simulink subsystem "LRLM_ECU"  (R2021a)
settings: Solver=VariableStepAuto  StartTime=0.0  StopTime=10.0  RelTol=1e-3
libraries: LRLM x4, simulink x2, BCM x1
settings Model: Creator=Sai229  LastModifiedBy=Sai229

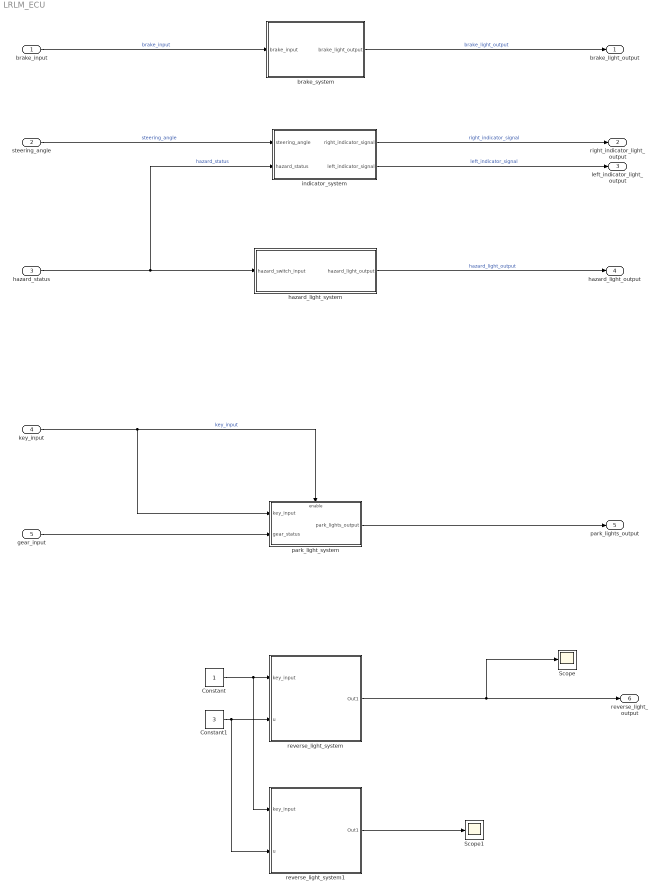
== system LRLM_ECU ==
  brake_input : Inport
  steering_angle : Inport  Port=2
  hazard_status : Inport  Port=3
  key_input : Inport  Port=4
  gear_input : Inport  Port=5
  Constant : Constant
  Constant1 : Constant  Value=3
  Scope : Scope
  Scope1 : Scope
  brake_system : Subsystem  TreatAsAtomicUnit=on
      mask Display: disp("Brake System");
  hazard_light_system : Subsystem
  indicator_system : Subsystem  TreatAsAtomicUnit=on
  park_light_system : Subsystem
  reverse_light_system : Subsystem  TreatAsAtomicUnit=on  mask{Parameter1=0, time_period=1}
      mask prompts: time_period "Enter the time period for blinking the light"
  reverse_light_system1 : Subsystem
      mask help: Simulink:masks:GenSFuncDesc_MD
      mask Help: eval('feval(''rtwprivate'',''rtwhelpview'',''rtw_sfcn_block'')');
  brake_light_output : Outport
  right_indicator_light_output : Outport  Port=2
  left_indicator_light_output : Outport  Port=3
  hazard_light_output : Outport  Port=4
  park_lights_output : Outport  Port=5
  reverse_light_output : Outport  Port=6
  wires:
  hazard_light_system/1(hazard_light_output) -> hazard_light_output/1  "hazard_light_output"
  brake_input/1 -> brake_system/1(brake_input)  "brake_input"
  park_light_system/1(park_lights_output) -> park_lights_output/1
  key_input/1 -> park_light_system/Enable, park_light_system/1(key_input)  "key_input"
  hazard_status/1 -> hazard_light_system/1(hazard_switch_input), indicator_system/2(hazard_status)  "hazard_status"
  indicator_system/2(left_indicator_signal) -> left_indicator_light_output/1  "left_indicator_signal"
  indicator_system/1(right_indicator_signal) -> right_indicator_light_output/1  "right_indicator_signal"
  steering_angle/1 -> indicator_system/1(steering_angle)  "steering_angle"
  brake_system/1(brake_light_output) -> brake_light_output/1  "brake_light_output"
  gear_input/1 -> park_light_system/2(gear_status)
  reverse_light_system/1(Out1) -> reverse_light_output/1, Scope/1
  reverse_light_system1/1(Out1) -> Scope1/1
  Constant/1 -> reverse_light_system/1(key_input), reverse_light_system1/1(key_input)
  Constant1/1 -> reverse_light_system/2(u), reverse_light_system1/2(u)

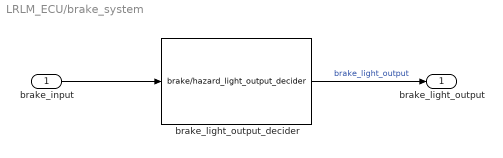
== system LRLM_ECU/brake_system ==
  brake_input : Inport
  brake_light_output_decider : LRLM/brake//hazard_light_output_decider
      settings: SourceProductName=LRLM Library
  brake_light_output : Outport
  wires:
  brake_light_output_decider/1 -> brake_light_output/1  "brake_light_output"
  brake_input/1 -> brake_light_output_decider/1

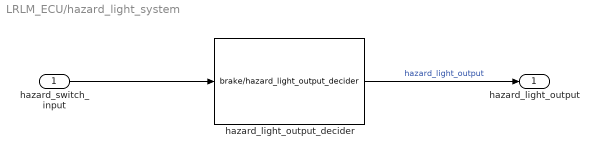
== system LRLM_ECU/hazard_light_system ==
  hazard_switch_input : Inport
  hazard_light_output_decider : LRLM/brake//hazard_light_output_decider
      settings: SourceProductName=LRLM Library
  hazard_light_output : Outport
  wires:
  hazard_light_output_decider/1 -> hazard_light_output/1  "hazard_light_output"
  hazard_switch_input/1 -> hazard_light_output_decider/1

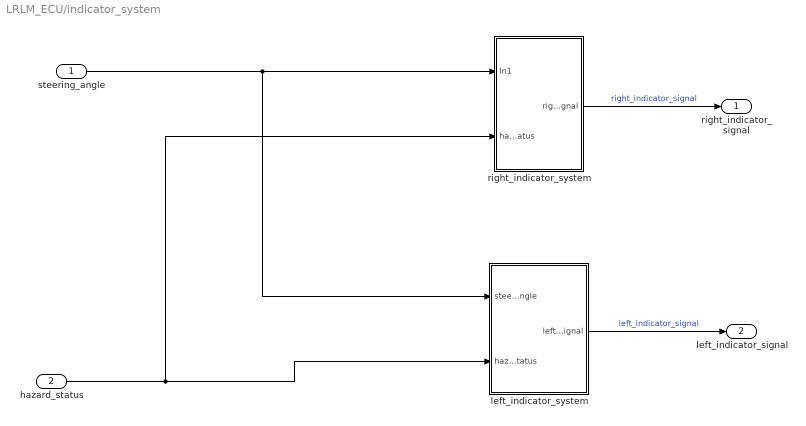
== system LRLM_ECU/indicator_system ==
  steering_angle : Inport
  hazard_status : Inport  Port=2
  left_indicator_system : Subsystem
  right_indicator_system : Subsystem
  right_indicator_signal : Outport
  left_indicator_signal : Outport  Port=2
  wires:
  steering_angle/1 -> right_indicator_system/1(In1), left_indicator_system/1(steering_angle)
  hazard_status/1 -> left_indicator_system/2(hazard_status), right_indicator_system/2(hazard_status)
  right_indicator_system/1(right_indicator_signal) -> right_indicator_signal/1  "right_indicator_signal"
  left_indicator_system/1(left_indicator_signal) -> left_indicator_signal/1  "left_indicator_signal"

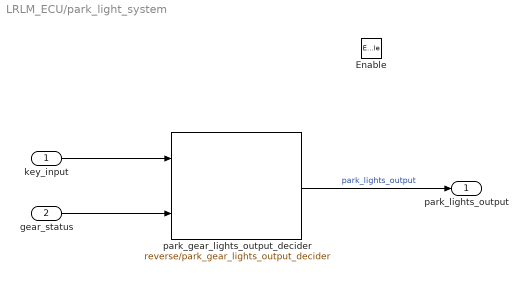
== system LRLM_ECU/park_light_system ==
  key_input : Inport
  gear_status : Inport  Port=2
  Enable : EnablePort  StatesWhenEnabling=reset
  park_gear_lights_output_decider : BCM/reverse//park_gear_lights_output_decider  gear_option=Park
      settings: SourceProductName=BCM Library
  park_lights_output : Outport
  wires:
  park_gear_lights_output_decider/1 -> park_lights_output/1  "park_lights_output"
  gear_status/1 -> park_gear_lights_output_decider/2
  key_input/1 -> park_gear_lights_output_decider/1

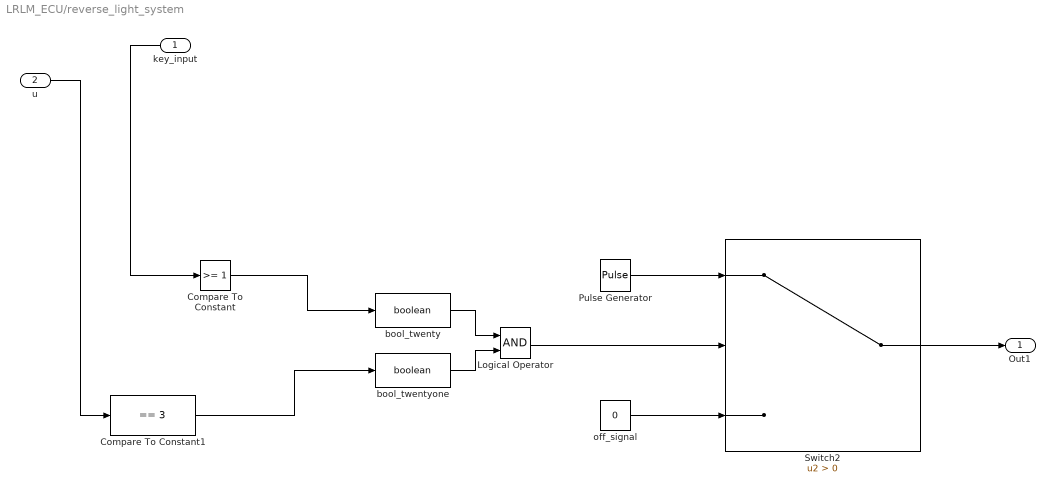
== system LRLM_ECU/reverse_light_system ==
  key_input : Inport
  u : Inport  Port=2
  Compare To Constant : simulink/Logic and Bit Operations/Compare To Constant  relop=>=  const=1  OutDataTypeStr=boolean
  Compare To Constant1 : simulink/Logic and Bit Operations/Compare To Constant  relop===  const=3  OutDataTypeStr=boolean
  Logical Operator : Logic  AllPortsSameDT=off  OutDataTypeStr=boolean
  Pulse Generator : DiscretePulseGenerator  PulseType=Time based  Amplitude=5  Period=time_period  PulseWidth=50
  Switch2 : Switch  Criteria=u2 > Threshold
  bool_twenty : DataTypeConversion  OutDataTypeStr=boolean
  bool_twentyone : DataTypeConversion  OutDataTypeStr=boolean
  off_signal : Constant  Value=0
  Out1 : Outport
  wires:
  u/1 -> Compare To Constant1/1
  Compare To Constant1/1 -> bool_twentyone/1
  Compare To Constant/1 -> bool_twenty/1
  key_input/1 -> Compare To Constant/1
  bool_twenty/1 -> Logical Operator/1
  Pulse Generator/1 -> Switch2/1
  off_signal/1 -> Switch2/3
  bool_twentyone/1 -> Logical Operator/2
  Logical Operator/1 -> Switch2/2
  Switch2/1 -> Out1/1

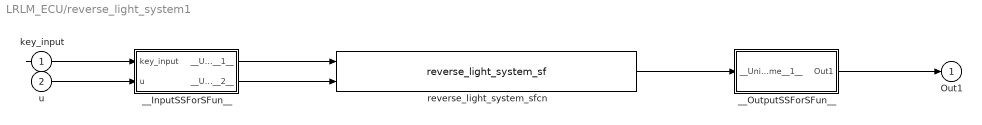
== system LRLM_ECU/reverse_light_system1 ==
  key_input : Inport
  u : Inport  Port=2
  __InputSSForSFun__ : Subsystem
  __OutputSSForSFun__ : Subsystem
  reverse_light_system_sfcn : S-Function  FunctionName=reverse_light_system_sf  SFunctionModules=""  SFunctionDeploymentMode=off  EnableBusSupport=off  mask{rtw_sf_name=reverse_light_system_sf, showVar=off}
      mask prompts: rtw_sf_name "Simulink:masks:GenSFuncName_MP"; showVar "Simulink:masks:GenSFuncShowModuleList_MP"
      mask help: Simulink:masks:GenSFuncDesc_MD
      mask init:
      | displist = '';
      | if ~strcmp(get_param(gcb, 'FunctionName'), rtw_sf_name);
      |   set_param(gcb, 'FunctionName', rtw_sf_name);
      | end
      | % Check if we are generating code
      | rtw_mode = false;
      | if strcmpi(get_param(bdroot(gcb),'SimulationStatus'),'Initializing')
      | 	rtw_mode = strcmpi(get_param(bdroot(gcb),'BuildingRTWCode'),'on') && ...
      | 		~strcmpi(get_param(bdroot(gcb),'TargetStyle'),'SimulationTarget');
      | end
      | if showVar || rtw_mode
      | 	if exist('rtwsfunc') == 2 | exist('rtwsfunc') == 6
      | 		tmplist = rtwsfunc(rtw_sf_name,gcb);
      | 		tmplist = DAStudio.message('Simulink:masks:GenSFuncListOfModules_IC', tmplist);
      | 	elseif showVar
      | 		tmplist1 = DAStudio.message('Simulink:masks:GenSFuncListOfModules_IC', '');
      |         tmplist2 = DAStudio.message('Simulink:masks:GenSFuncNotLicensed_IC');
      |         tmplist = [tmplist1 tmplist2];
      |  	end
      | end
      | if showVar
      |   displist = tmplist;
      | end
      settings: CopyFcn=|
      | if ~strcmp(get_param(gcb,'Linkstatus'),'none') && ...
      | ~strcmp(get_param(gcb,'Linkstatus'),'implicit')
      |   set_param(gcb,'LinkStatus','none');
      | end
      mask Help: eval('feval(''rtwprivate'',''rtwhelpview'',''rtw_sfcn_block'')');
      mask DialogControl rtw_sf_name Prompt: Generated S-function name (model_sf):
      mask DialogControl showVar Prompt: Show module list
      mask Display:
      | port_label('input',1,'key_input');
      | port_label('input',2,'u');
      | port_label('output',1,'Out1');
  Out1 : Outport
  wires:
  __OutputSSForSFun__/1(Out1) -> Out1/1
  reverse_light_system_sfcn/1 -> __OutputSSForSFun__/1(__UniqueInportName__1__)
  __InputSSForSFun__/2(__UniqueOutportName__2__) -> reverse_light_system_sfcn/2
  __InputSSForSFun__/1(__UniqueOutportName__1__) -> reverse_light_system_sfcn/1
  u/1 -> __InputSSForSFun__/2(u)
  key_input/1 -> __InputSSForSFun__/1(key_input)

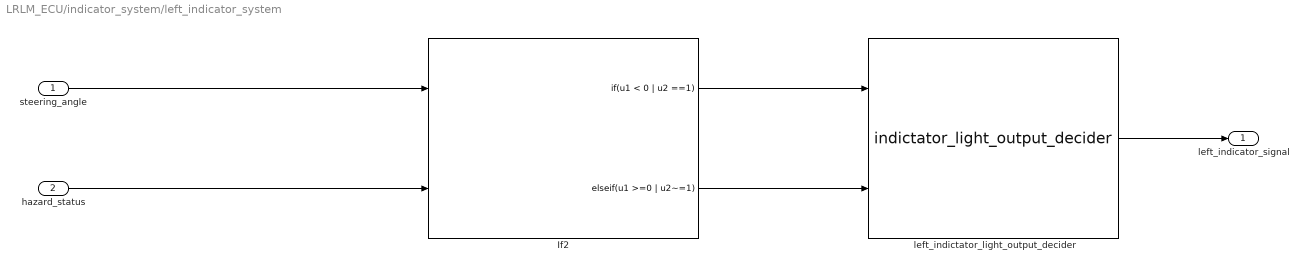
== system LRLM_ECU/indicator_system/left_indicator_system ==
  steering_angle : Inport
  hazard_status : Inport  Port=2
  If2 : If  NumInputs=2  IfExpression=u1 < 0 | u2 ==1  ElseIfExpressions=u1 >=0 | u2~=1  ShowElse=off
  left_indictator_light_output_decider : LRLM/indictator_light_output_decider
      settings: SourceProductName=LRLM Library
  left_indicator_signal : Outport
  wires:
  left_indictator_light_output_decider/1 -> left_indicator_signal/1
  If2/2 -> left_indictator_light_output_decider/2
  If2/1 -> left_indictator_light_output_decider/1
  steering_angle/1 -> If2/1
  hazard_status/1 -> If2/2

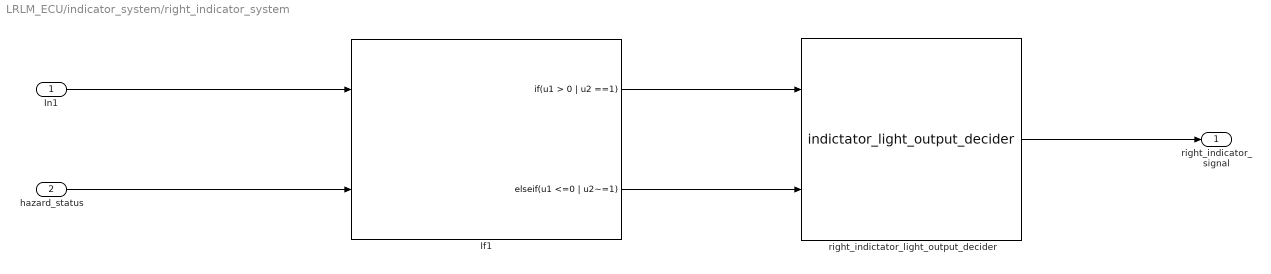
== system LRLM_ECU/indicator_system/right_indicator_system ==
  In1 : Inport
  hazard_status : Inport  Port=2
  If1 : If  NumInputs=2  IfExpression=u1 > 0 | u2 ==1  ElseIfExpressions=u1 <=0 | u2~=1  ShowElse=off
  right_indictator_light_output_decider : LRLM/indictator_light_output_decider
      settings: SourceProductName=LRLM Library
  right_indicator_signal : Outport
  wires:
  right_indictator_light_output_decider/1 -> right_indicator_signal/1
  If1/2 -> right_indictator_light_output_decider/2
  If1/1 -> right_indictator_light_output_decider/1
  In1/1 -> If1/1
  hazard_status/1 -> If1/2

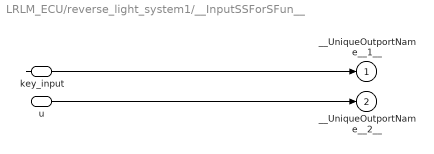
== system LRLM_ECU/reverse_light_system1/__InputSSForSFun__ ==
  key_input : Inport
  u : Inport  Port=2
  __UniqueOutportName__1__ : Outport
  __UniqueOutportName__2__ : Outport  Port=2
  wires:
  u/1 -> __UniqueOutportName__2__/1
  key_input/1 -> __UniqueOutportName__1__/1

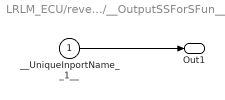
== system LRLM_ECU/reverse_light_system1/__OutputSSForSFun__ ==
  __UniqueInportName__1__ : Inport
  Out1 : Outport
  wires:
  __UniqueInportName__1__/1 -> Out1/1
